simulink model "simulink_model_3_task"  (R2021b)
settings: Solver=FixedStepAuto  StartTime=0.0  StopTime=0.03  FixedStep=0.0001  RelTol=1e-3
model workspace (MAT data in the model file):
  Ia = 0
  Ia_var = 0
  Ib = 0
  Ib_var = 0
  Ya = 0.5
  Ya_var = 0.5
  Yb = 0.5
  Yb_var = 0.5
  w = 100
  w_var = 0
settings Model: Creator=mluser  LastModifiedBy=alisheryuldashov
settings SolverCC: AlgebraicLoopSolver=TrustRegion
settings DebuggingCC: UnconnectedInputMsg=none  UnconnectedOutputMsg=none  UnconnectedLineMsg=none  ArithmeticOperatorsInVariantConditions=warning
settings SFSimCC: CustomCodeUndefinedFunction=UseInterfaceOnly
settings CodeAppCC: StateflowObjectComments=on

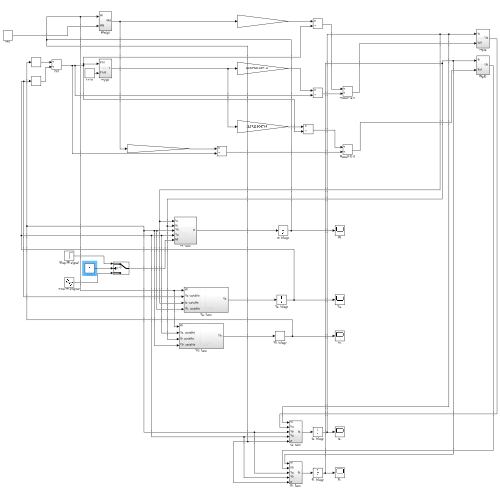
[thumbnail: Simulink's stored preview of the top-level diagram]
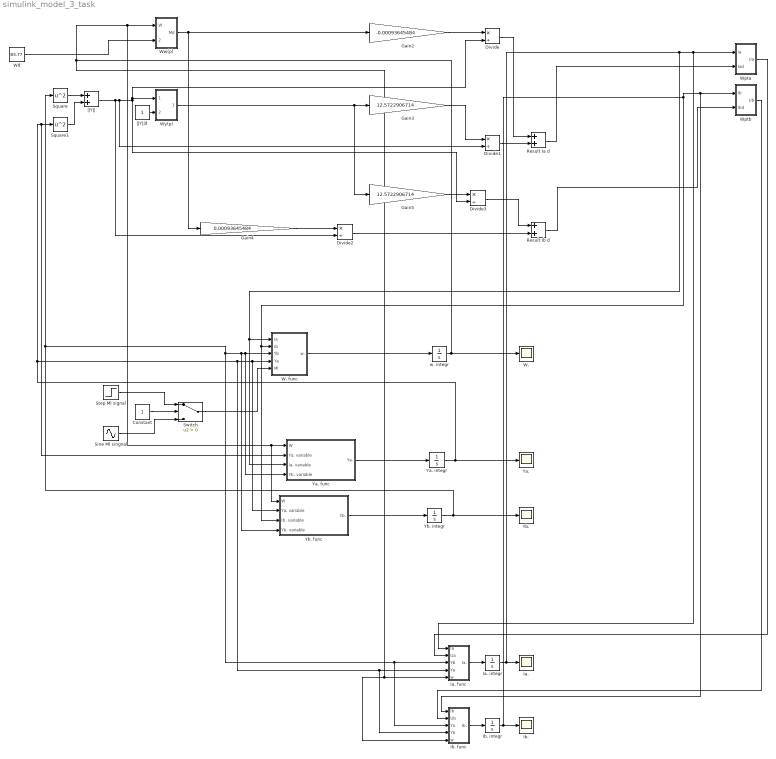
== system simulink_model_3_task ==
  Constant : Constant
  Divide{,1..3} (4 alike) : Product  Inputs=*/
  Gain2 : Gain  Gain=-0.00093645484
  Gain3 : Gain  Gain=12.5722906714
  Gain4 : Gain  Gain=0.00093645484
  Gain5 : Gain  Gain=12.5722906714
  Ia. : Scope
  Ia. func : Subsystem
  Ia. integr : Integrator  InitialCondition=Ia_var
  Ib. : Scope
  Ib. func : Subsystem
  Ib. integr : Integrator  InitialCondition=Ib_var
  Result Ia d : Sum
  Result Ib d : Sum
  Sine Ml singnal : Sin  Amplitude=83.9389490944  SampleTime=0
  Square : Math  Operator=square  SignedPower=on  SaturateOnIntegerOverflow=on
  Square1 : Math  Operator=square  SignedPower=on  SaturateOnIntegerOverflow=on
  Step Ml signal : Step  After=83.9389490944  SampleTime=0
  Switch : Switch  Criteria=u2 > Threshold
  W. : Scope
  W. func : Subsystem
  Wd : Constant  Value=83.77
  Wpta : Subsystem
  Wptb : Subsystem
  Ww(p) : Subsystem
  Wy(p) : Subsystem
  Ya. : Scope
  Ya. func : Subsystem
  Ya. integr : Integrator  InitialCondition=Ya_var
  Yb. : Scope
  Yb. func : Subsystem
  Yb. integr : Integrator  InitialCondition=Yb_var
  w. integr : Integrator  InitialCondition=w_var
  ||Y|| : Sum
  ||Y||d : Constant
  wires:
  Ya. integr/1 -> Ya./1, Ya. func/2(Ya. variable), Square1/1, Ib. func/4(Yb), Ia. func/4(Ya), Yb. func/2(Ya. variable), W. func/4(Ya)
  Square/1 -> ||Y||/1
  Square1/1 -> ||Y||/2
  ||Y||/1 -> Divide2/2, Divide1/2, Wy(p)/1(||Y||), Divide/2, Divide3/2
  Gain2/1 -> Divide/1
  Gain3/1 -> Divide1/1
  Divide/1 -> Result Ia d/1
  Divide1/1 -> Result Ia d/2
  Result Ia d/1 -> Wpta/2(Iad)
  Gain4/1 -> Divide2/1
  Gain5/1 -> Divide3/1
  Divide3/1 -> Result Ib d/1
  Divide2/1 -> Result Ib d/2
  Result Ib d/1 -> Wptb/2(Ibd)
  Step Ml signal/1 -> Switch/1
  Sine Ml singnal/1 -> Switch/3
  Constant/1 -> Switch/2
  Ww(p)/1(Md) -> Gain2/1, Gain4/1
  w. integr/1 -> W./1, Yb. func/1(W), Ya. func/1(W), Ww(p)/1(W), Ib. func/5(w), Ia. func/5(w)
  Wd/1 -> Ww(p)/2(Wd)
  Wy(p)/1(Out1) -> Gain5/1, Gain3/1
  ||Y||d/1 -> Wy(p)/2(||Yd||)
  Ia. integr/1 -> Ya. func/3(Ia. variable), W. func/1(Ia), Ia. func/1(Ia), Wpta/1(Ia), Ia./1
  Ib. integr/1 -> Ib./1, Ib. func/1(Ib), Wptb/1(Ib), Yb. func/3(Ib. variable), W. func/2(Ib)
  Switch/1 -> W. func/5(Ml)
  Yb. integr/1 -> Yb./1, Square/1, Ib. func/3(Ya), Ia. func/3(Yb), Yb. func/4(Yb. variable), Ya. func/4(Yb. variable), W. func/3(Yb)
  Wpta/1(Ua) -> Ia. func/2(Ua)
  Wptb/1(Ub) -> Ib. func/2(Ub)
  Ya. func/1(Ya.) -> Ya. integr/1
  W. func/1(w.) -> w. integr/1
  Yb. func/1(Yb.) -> Yb. integr/1
  Ib. func/1(Ib.) -> Ib. integr/1
  Ia. func/1(Ia.) -> Ia. integr/1

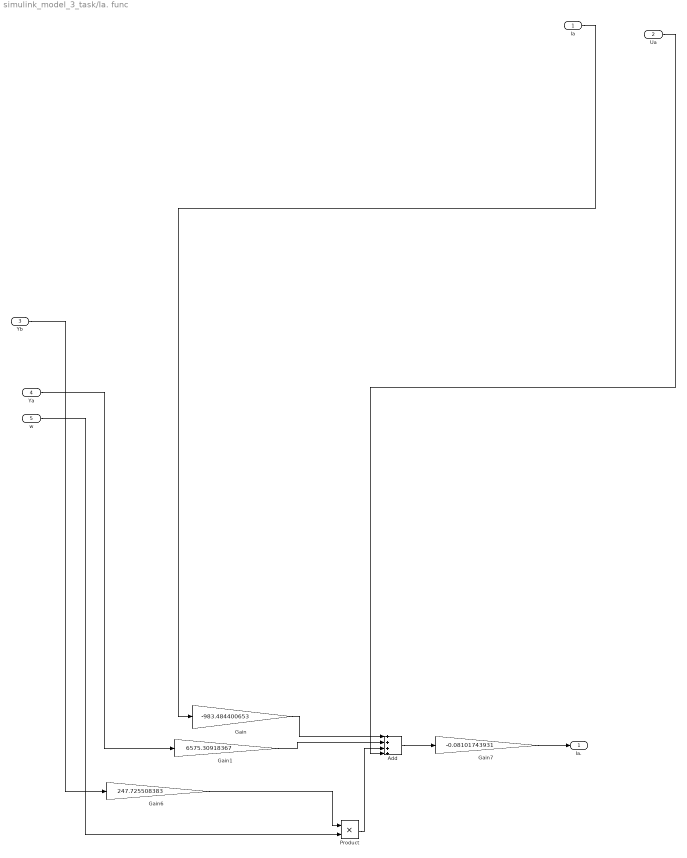
== system simulink_model_3_task/Ia. func ==
  Ia : Inport
  Ua : Inport  Port=2
  Yb : Inport  Port=3
  Ya : Inport  Port=4
  w : Inport  Port=5
  Add : Sum  Inputs=++++
  Gain : Gain  Gain=-983.484400653
  Gain1 : Gain  Gain=6575.30918367
  Gain6 : Gain  Gain=247.725508383
  Gain7 : Gain  Gain=-0.08101743931
  Product : Product
  Ia. : Outport
  wires:
  Ua/1 -> Add/4
  Yb/1 -> Gain6/1
  Gain7/1 -> Ia./1
  Product/1 -> Add/3
  Gain/1 -> Add/1
  Ia/1 -> Gain/1
  Gain1/1 -> Add/2
  Add/1 -> Gain7/1
  Ya/1 -> Gain1/1
  w/1 -> Product/2
  Gain6/1 -> Product/1

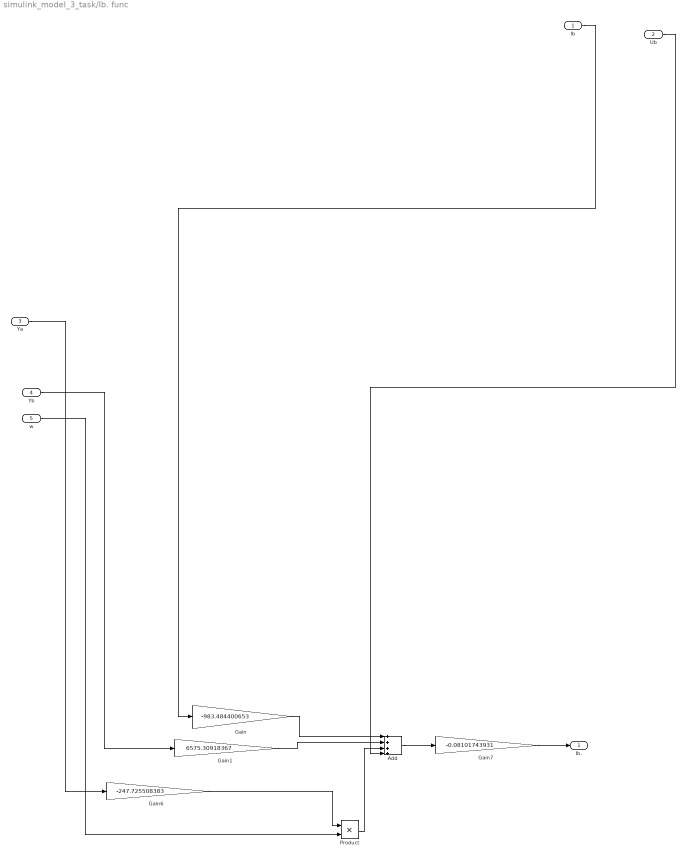
== system simulink_model_3_task/Ib. func ==
  Ib : Inport
  Ub : Inport  Port=2
  Ya : Inport  Port=3
  Yb : Inport  Port=4
  w : Inport  Port=5
  Add : Sum  Inputs=++++
  Gain : Gain  Gain=-983.484400653
  Gain1 : Gain  Gain=6575.30918367
  Gain6 : Gain  Gain=-247.725508383
  Gain7 : Gain  Gain=-0.08101743931
  Product : Product
  Ib. : Outport
  wires:
  Ub/1 -> Add/4
  Ya/1 -> Gain6/1
  Gain7/1 -> Ib./1
  Product/1 -> Add/3
  Gain/1 -> Add/1
  Ib/1 -> Gain/1
  Gain1/1 -> Add/2
  Add/1 -> Gain7/1
  Yb/1 -> Gain1/1
  w/1 -> Product/2
  Gain6/1 -> Product/1

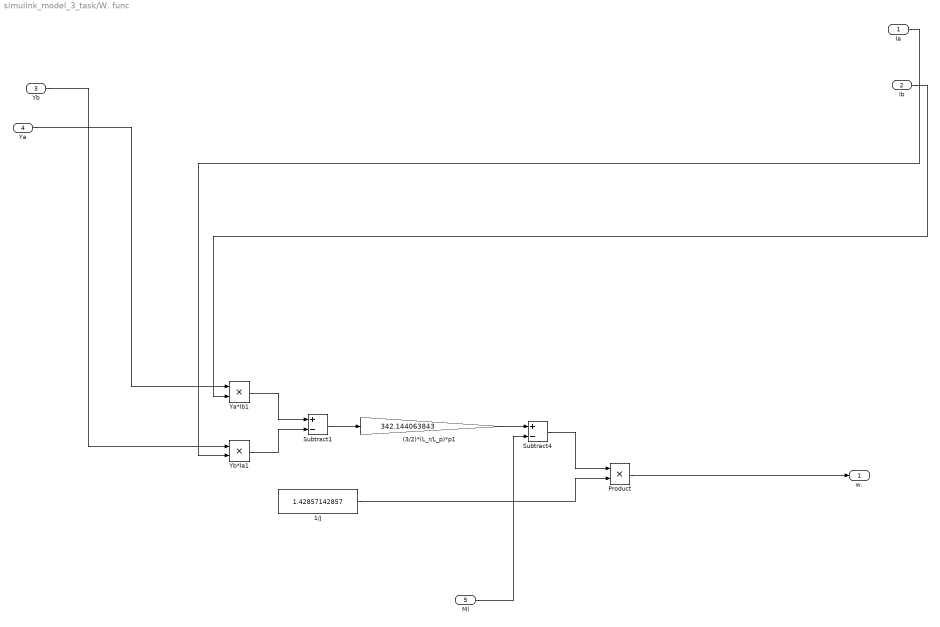
== system simulink_model_3_task/W. func ==
  Ia : Inport
  Ib : Inport  Port=2
  Yb : Inport  Port=3
  Ya : Inport  Port=4
  Ml : Inport  Port=5
  (3/2)*(L_r/L_p)*p1 : Gain  Gain=342.144063843
  1/J : Constant  Value=1.42857142857
  Product : Product
  Subtract1 : Sum  Inputs=+-
  Subtract4 : Sum  Inputs=+-
  Ya*Ib1 : Product
  Yb*Ia1 : Product
  w. : Outport
  wires:
  Ml/1 -> Subtract4/2
  Product/1 -> w./1
  1/J/1 -> Product/2
  Subtract1/1 -> (3/2)*(L_r/L_p)*p1/1
  Yb/1 -> Yb*Ia1/1
  Ya*Ib1/1 -> Subtract1/1
  Yb*Ia1/1 -> Subtract1/2
  Ia/1 -> Yb*Ia1/2
  Ya/1 -> Ya*Ib1/1
  Ib/1 -> Ya*Ib1/2
  (3/2)*(L_r/L_p)*p1/1 -> Subtract4/1
  Subtract4/1 -> Product/1

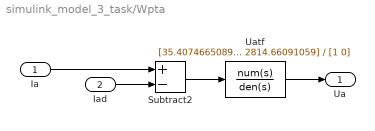
== system simulink_model_3_task/Wpta ==
  Ia : Inport
  Iad : Inport  Port=2
  Subtract2 : Sum  Inputs=+-
  Uatf : TransferFcn  Numerator=[35.4074665089 2814.66091059]  Denominator=[1 0]
  Ua : Outport
  wires:
  Ia/1 -> Subtract2/1
  Iad/1 -> Subtract2/2
  Uatf/1 -> Ua/1
  Subtract2/1 -> Uatf/1

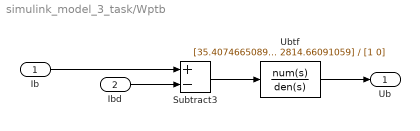
== system simulink_model_3_task/Wptb ==
  Ib : Inport
  Ibd : Inport  Port=2
  Subtract3 : Sum  Inputs=+-
  Ubtf : TransferFcn  Numerator=[35.4074665089 2814.66091059]  Denominator=[1 0]
  Ub : Outport
  wires:
  Ib/1 -> Subtract3/1
  Ibd/1 -> Subtract3/2
  Ubtf/1 -> Ub/1
  Subtract3/1 -> Ubtf/1

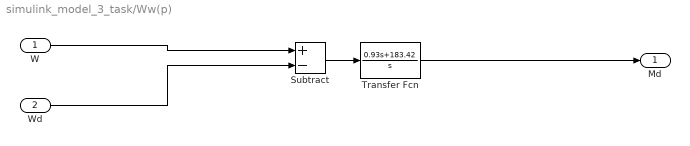
== system simulink_model_3_task/Ww(p) ==
  W : Inport
  Wd : Inport  Port=2
  Subtract : Sum  Inputs=+-
  Transfer Fcn : TransferFcn  Numerator=[0.93 183.42]  Denominator=[1 0]
  Md : Outport
  wires:
  Transfer Fcn/1 -> Md/1
  W/1 -> Subtract/1
  Wd/1 -> Subtract/2
  Subtract/1 -> Transfer Fcn/1

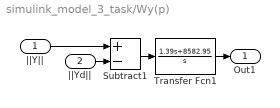
== system simulink_model_3_task/Wy(p) ==
  ||Y|| : Inport
  ||Yd|| : Inport  Port=2
  Subtract1 : Sum  Inputs=+-
  Transfer Fcn1 : TransferFcn  Numerator=[1.39 8582.95]  Denominator=[1 0]
  Out1 : Outport
  wires:
  ||Yd||/1 -> Subtract1/2
  ||Y||/1 -> Subtract1/1
  Transfer Fcn1/1 -> Out1/1
  Subtract1/1 -> Transfer Fcn1/1

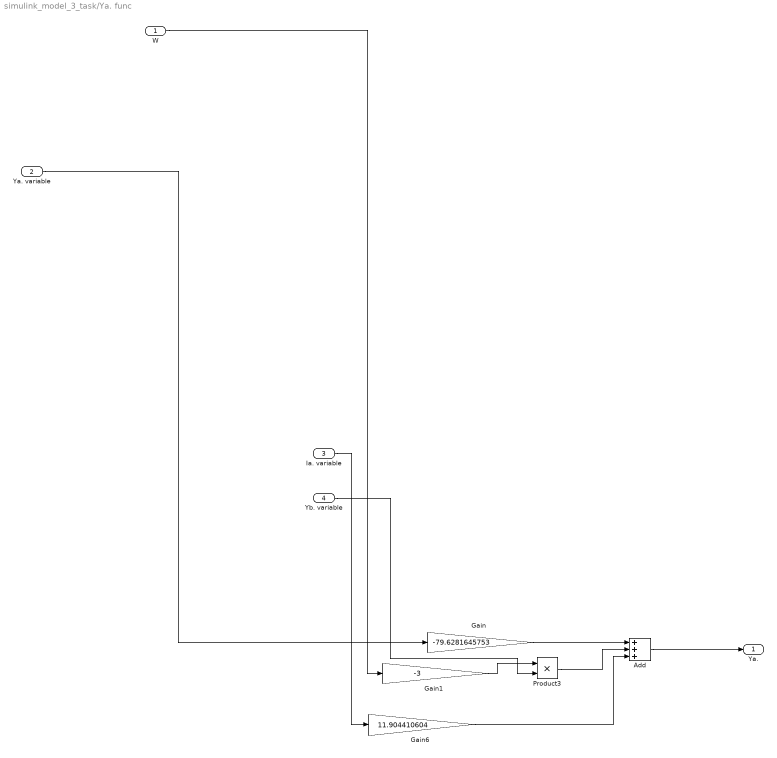
== system simulink_model_3_task/Ya. func ==
  W : Inport
  Ya. variable : Inport  Port=2
  Ia. variable : Inport  Port=3
  Yb. variable : Inport  Port=4
  Add : Sum  Inputs=+++
  Gain : Gain  Gain=-79.6281645753
  Gain1 : Gain  Gain=-3
  Gain6 : Gain  Gain=11.904410604
  Product3 : Product
  Ya. : Outport
  wires:
  Yb. variable/1 -> Product3/2
  W/1 -> Gain1/1
  Add/1 -> Ya./1
  Gain1/1 -> Product3/1
  Ya. variable/1 -> Gain/1
  Gain/1 -> Add/1
  Gain6/1 -> Add/3
  Ia. variable/1 -> Gain6/1
  Product3/1 -> Add/2

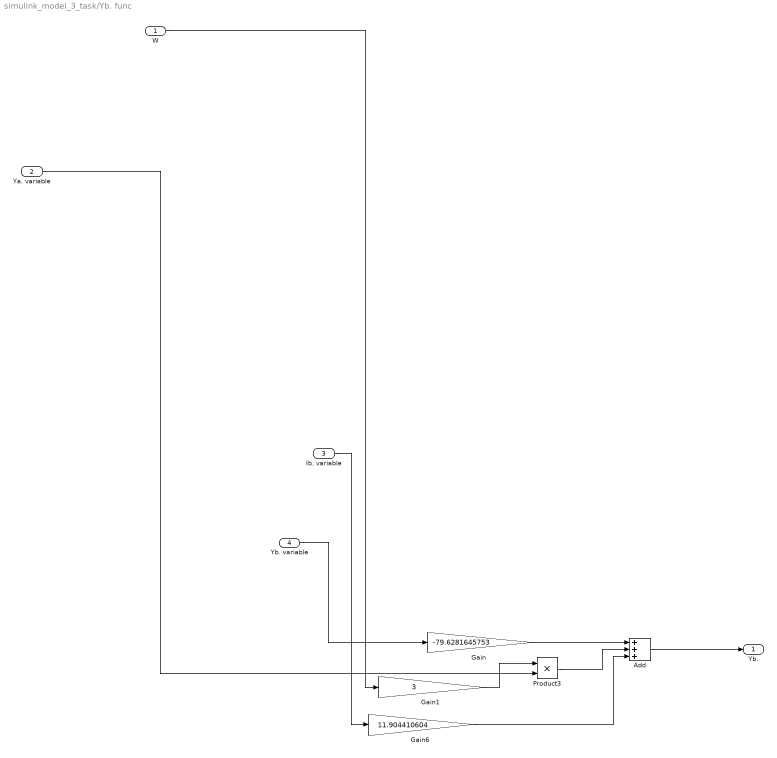
== system simulink_model_3_task/Yb. func ==
  W : Inport
  Ya. variable : Inport  Port=2
  Ib. variable : Inport  Port=3
  Yb. variable : Inport  Port=4
  Add : Sum  Inputs=+++
  Gain : Gain  Gain=-79.6281645753
  Gain1 : Gain  Gain=3
  Gain6 : Gain  Gain=11.904410604
  Product3 : Product
  Yb. : Outport
  wires:
  W/1 -> Gain1/1
  Add/1 -> Yb./1
  Gain1/1 -> Product3/1
  Gain/1 -> Add/1
  Gain6/1 -> Add/3
  Ib. variable/1 -> Gain6/1
  Product3/1 -> Add/2
  Ya. variable/1 -> Product3/2
  Yb. variable/1 -> Gain/1
